simulink model "ModelDosingUnit"  (R2020b)
settings: Solver=FixedStepAuto  StartTime=0.0  StopTime=1  FixedStep=0.010  RelTol=1e-3
settings Model: Creator=kaebi  LastModifiedBy=kaebi
settings OptimizationCC: DefaultParameterBehavior=Inlined  LocalBlockOutputs=off
settings RTWCC: Description=TwinCAT GRT Target  SystemTargetFile=TwinCatGrt.tlc  GenCodeOnly=on  TemplateMakefile=tcgrt_msbuild.tmf  TargetLang=C++
settings STFCustomTargetCC: TargetLangStandard=C++03 (ISO)  ConcurrentExecutionCompliant=off  CombineOutputUpdateFcns=on  CodeInterfacePackaging=Reusable function  GRTInterface=off  GenerateAllocFcn=on  SystemTargetFile=TwinCatGrt.tlc
settings GRTTargetCC: TargetLangStandard=C++03 (ISO)  ParMdlRefBuildCompliant=off  CompOptLevelCompliant=off  ConcurrentExecutionCompliant=off  MatFileLogging=off  CodeInterfacePackaging=Reusable function  GenerateAllocFcn=on  UseToolchainInfoCompliant=off  ExtModeMexFile=TcExtModeClient

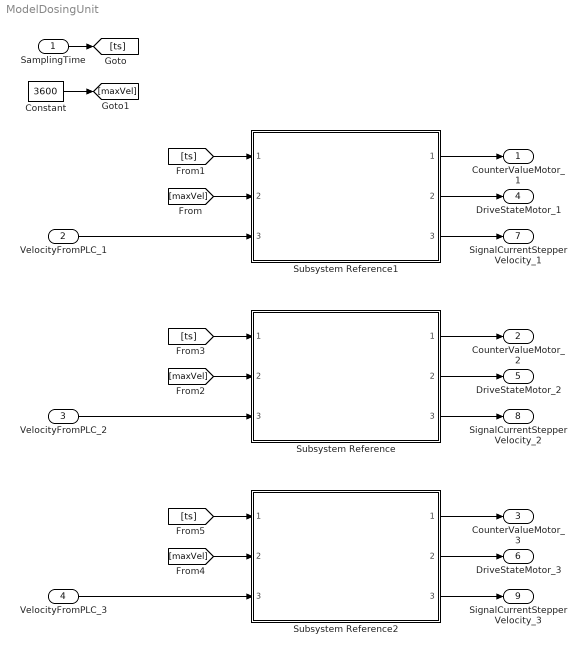
== system ModelDosingUnit ==
  SamplingTime : Inport
  VelocityFromPLC_1 : Inport  Port=2  OutDataTypeStr=int16
  VelocityFromPLC_2 : Inport  Port=3  OutDataTypeStr=int16
  VelocityFromPLC_3 : Inport  Port=4  OutDataTypeStr=int16
  Constant : Constant  Value=3600
  Subsystem Reference : Subsystem  ReferencedSubsystem=SubsystemGenericDrive
  Subsystem Reference1 : Subsystem  ReferencedSubsystem=SubsystemGenericDrive
  Subsystem Reference2 : Subsystem  ReferencedSubsystem=SubsystemGenericDrive
  CounterValueMotor_1 : Outport  OutDataTypeStr=uint16
  CounterValueMotor_2 : Outport  Port=2  OutDataTypeStr=uint16
  CounterValueMotor_3 : Outport  Port=3  OutDataTypeStr=uint16
  DriveStateMotor_1 : Outport  Port=4  OutDataTypeStr=uint8
  DriveStateMotor_2 : Outport  Port=5  OutDataTypeStr=uint8
  DriveStateMotor_3 : Outport  Port=6  OutDataTypeStr=uint8
  SignalCurrentStepperVelocity_1 : Outport  Port=7
  SignalCurrentStepperVelocity_2 : Outport  Port=8
  SignalCurrentStepperVelocity_3 : Outport  Port=9
  wires:
  SamplingTime/1 -> [ts]
  Constant/1 -> [maxVel]
  [ts] -> Subsystem Reference1/1
  VelocityFromPLC_1/1 -> Subsystem Reference1/3
  [maxVel] -> Subsystem Reference1/2
  Subsystem Reference1/1 -> CounterValueMotor_1/1
  Subsystem Reference1/2 -> DriveStateMotor_1/1
  Subsystem Reference1/3 -> SignalCurrentStepperVelocity_1/1
  Subsystem Reference/3 -> SignalCurrentStepperVelocity_2/1
  Subsystem Reference/2 -> DriveStateMotor_2/1
  Subsystem Reference/1 -> CounterValueMotor_2/1
  [maxVel] -> Subsystem Reference/2
  VelocityFromPLC_2/1 -> Subsystem Reference/3
  [ts] -> Subsystem Reference/1
  [ts] -> Subsystem Reference2/1
  VelocityFromPLC_3/1 -> Subsystem Reference2/3
  [maxVel] -> Subsystem Reference2/2
  Subsystem Reference2/1 -> CounterValueMotor_3/1
  Subsystem Reference2/2 -> DriveStateMotor_3/1
  Subsystem Reference2/3 -> SignalCurrentStepperVelocity_3/1
